simulink model "class_3_simulink"  (R2023b)
settings: Solver=VariableStepAuto  StartTime=0.0  StopTime=10.0  RelTol=1e-3
undefined symbols (not defined in the file): A, B, denp, h, I, K, kr, nump, s
libraries: cstblocks x4
settings Model: Creator=klysm  LastModifiedBy=klysm

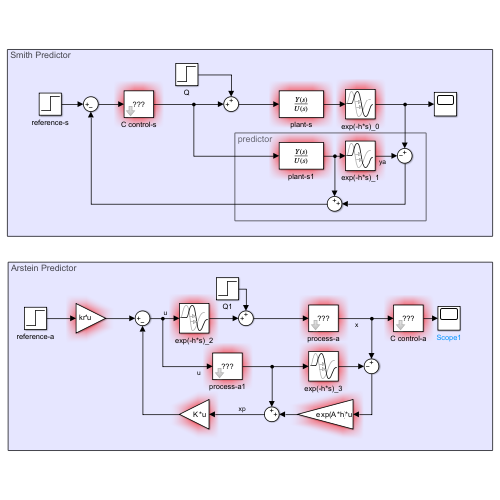
[thumbnail: Simulink's stored preview of the top-level diagram]
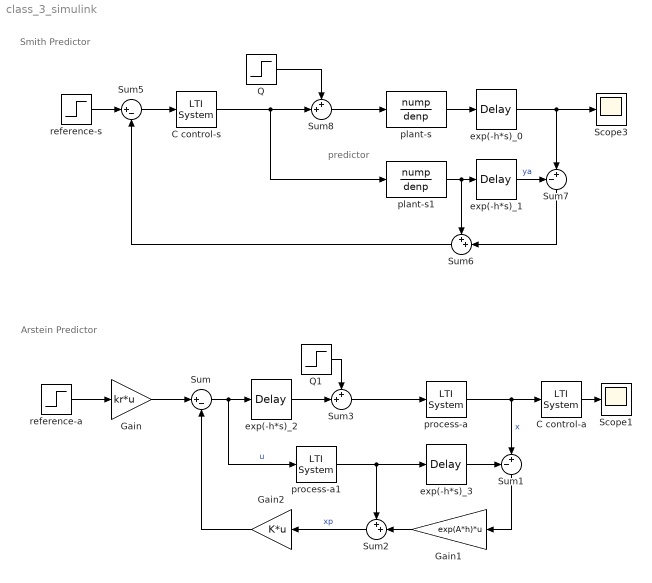
== system class_3_simulink ==
  note: predictor
  note: Arstein Predictor
  note: Smith Predictor
  C control-a : cstblocks/LTI System  sys=C  IC=[]  PadeOrder=0
  C control-s : cstblocks/LTI System  sys=C  IC=[]  PadeOrder=0
  Gain : Gain  Gain=kr*u
  Gain1 : Gain  Gain=exp(A*h)*u
  Gain2 : Gain  Gain=K*u
  Q : Step  SampleTime=0
  Q1 : Step  SampleTime=0
  Scope1 : Scope
  Scope3 : Scope
  Sum : Sum  Inputs=|+-
  Sum1 : Sum  Inputs=-+|
  Sum{2..3,6,8} (4 alike) : Sum  Inputs=++|
  Sum5 : Sum  Inputs=|+-
  Sum7 : Sum  Inputs=-+|
  exp(-h*s)_{0..3} (4 alike) : TransportDelay  DelayTime=h
  plant-s : TransferFcn  Numerator=nump  Denominator=denp
  plant-s1 : TransferFcn  Numerator=nump  Denominator=denp
  process-a : cstblocks/LTI System  sys=inv(s*I-A)*B  IC=[]  PadeOrder=0
  process-a1 : cstblocks/LTI System  sys=inv(s*I-A)*B  IC=[]  PadeOrder=0
  reference-a : Step  SampleTime=0
  reference-s : Step  SampleTime=0
  wires:
  Sum8/1 -> plant-s/1
  Q/1 -> Sum8/1
  exp(-h*s)_0/1 -> Scope3/1, Sum7/2
  exp(-h*s)_1/1 -> Sum7/1  "ya"
  plant-s1/1 -> Sum6/1, exp(-h*s)_1/1
  reference-s/1 -> Sum5/1
  C control-s/1 -> Sum8/2, plant-s1/1
  Sum6/1 -> Sum5/2
  Sum5/1 -> C control-s/1
  Sum7/1 -> Sum6/2
  plant-s/1 -> exp(-h*s)_0/1
  Gain/1 -> Sum/1
  reference-a/1 -> Gain/1
  Sum/1 -> process-a1/1, exp(-h*s)_2/1  "u"
  exp(-h*s)_2/1 -> Sum3/2
  process-a1/1 -> exp(-h*s)_3/1, Sum2/1
  process-a/1 -> C control-a/1, Sum1/2  "x"
  exp(-h*s)_3/1 -> Sum1/1
  C control-a/1 -> Scope1/1
  Gain1/1 -> Sum2/2
  Sum1/1 -> Gain1/1
  Sum2/1 -> Gain2/1  "xp"
  Gain2/1 -> Sum/2
  Sum3/1 -> process-a/1
  Q1/1 -> Sum3/1
